simulink model "SixDsimulator_M1B"  (R2021a)
settings: Solver=FixedStepDiscrete  StartTime=0.0  StopTime=200  FixedStep=.1  RelTol=1e-3
libraries: simulink x1
settings Model: Creator=tranka  LastModifiedBy=tranka

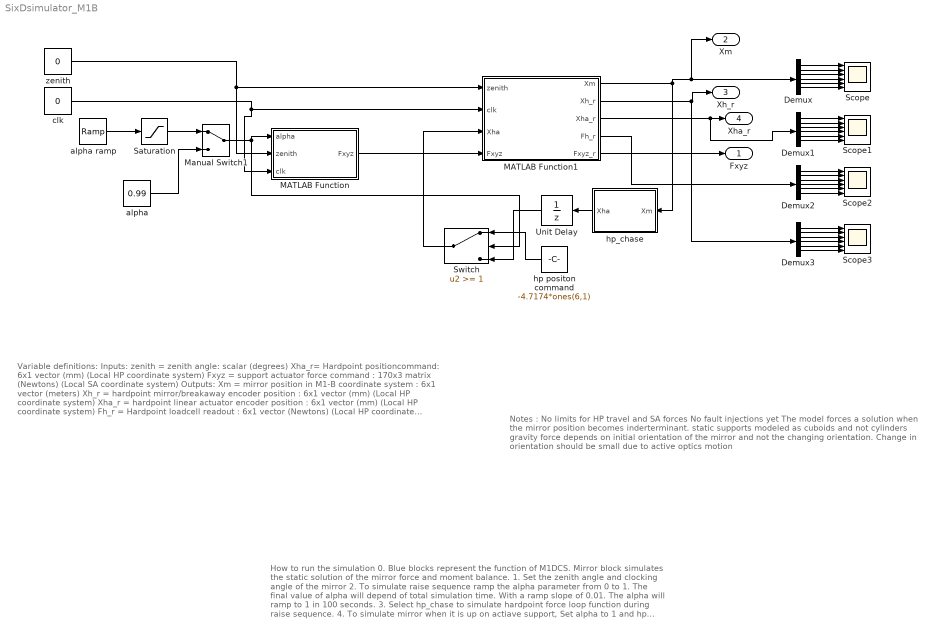
== system SixDsimulator_M1B ==
  note: How to run the simulation
      |
      | 0. Blue blocks represent the function of M1DCS. Mirror block simulates the static solution of the mirror force and moment balance.
      | 1. Set the zenith angle and clocking angle of the mirror
      | 2. To simulate raise sequence ramp the alpha parameter from 0 to 1. The final value of alpha will depend of total simulation time. With a ramp slope of 0.01. The alpha will ramp to 1 in 100 seconds.
      | 3. Select hp_chase to simulate hardpoint force loop function during raise sequence.
      | 4. To simulate mirror when it is up on actiave support, Set alpha to 1 and hp position command as user input.
  note: Variable definitions:
      |
      | Inputs:
      | zenith = zenith angle: scalar (degrees)
      | Xha_r= Hardpoint positioncommand: 6x1 vector (mm) (Local HP coordinate system)
      | Fxyz = support actuator force command : 170x3 matrix (Newtons) (Local SA coordinate system)
      |
      | Outputs:
      | Xm = mirror position in M1-B coordinate system : 6x1 vector (meters)
      | Xh_r = hardpoint mirror/breakaway encoder position : 6x1 vector (mm) (Local HP coordinate system)
      | Xha_r = hardpoint linear actuator encoder position : 6x1 vector (mm) (Local HP coordinate system)
      | Fh_r = Hardpoint loadcell readout : 6x1 vector (Newtons) (Local HP coordinate system)
      | FXYZ_r = support actuator force readback : 170x3 matrix (SA local coordinate system)
  note: Notes :
      |
      | No limits for HP travel and SA forces
      | No fault injections yet
      | The model forces a solution when the mirror position becomes inderterminant.
      | static supports modeled as cuboids and not cylinders
      | gravity force depends on initial orientation of the mirror and not the changing orientation.
      | Change in orientation should be small due to active optics motion
  Demux{,1..3} (4 alike) : Demux  Outputs=6
  MATLAB Function : MATLAB Function  TreatAsAtomicUnit=on
  MATLAB Function1 : MATLAB Function  TreatAsAtomicUnit=on
  Manual Switch1 : ManualSwitch
  Saturation : Saturate  UpperLimit=1  LowerLimit=-1
  Scope{,1..3} (4 alike) : Scope  NumInputPorts=6
  Switch : Switch  Threshold=1
  Unit Delay : UnitDelay  SampleTime=-1  HasFrameUpgradeWarning=on
  alpha : Constant  Value=0.99
  alpha ramp : simulink/Sources/Ramp  slope=0.01  start=0  InitialOutput=0
  clk : Constant  Value=0
  hp positon command : Constant  Value=-4.7174*ones(6,1)
  hp_chase : MATLAB Function  TreatAsAtomicUnit=on
  zenith : Constant  Value=0
  Fxyz : Outport
  Xm : Outport  Port=2
  Xh_r : Outport  Port=3
  Xha_r : Outport  Port=4
  wires:
  MATLAB Function/1(Fxyz) -> MATLAB Function1/4(Fxyz)
  zenith/1 -> MATLAB Function1/1(zenith), MATLAB Function/2(zenith)
  MATLAB Function1/1(Xm) -> Xm/1, Demux/1, hp_chase/1(Xm)
  hp_chase/1(Xha) -> Unit Delay/1
  Demux/3 -> Scope/3
  Demux/4 -> Scope/4
  Demux/5 -> Scope/5
  Demux/2 -> Scope/2
  Demux/6 -> Scope/6
  Demux/1 -> Scope/1
  Demux1/1 -> Scope1/1
  Demux1/2 -> Scope1/2
  Demux1/3 -> Scope1/3
  Demux1/4 -> Scope1/4
  Demux1/5 -> Scope1/5
  Demux1/6 -> Scope1/6
  MATLAB Function1/3(Xha_r) -> Demux1/1, Xha_r/1
  Demux2/1 -> Scope2/1
  Demux2/2 -> Scope2/2
  Demux2/3 -> Scope2/3
  Demux2/5 -> Scope2/5
  Demux2/6 -> Scope2/6
  Demux2/4 -> Scope2/4
  MATLAB Function1/4(Fh_r) -> Demux2/1
  alpha ramp/1 -> Saturation/1
  alpha/1 -> Manual Switch1/2
  Manual Switch1/1 -> Switch/2, MATLAB Function/1(alpha)
  clk/1 -> MATLAB Function/3(clk), MATLAB Function1/2(clk)
  MATLAB Function1/5(Fxyz_r) -> Fxyz/1
  MATLAB Function1/2(Xh_r) -> Demux3/1, Xh_r/1
  Demux3/1 -> Scope3/1
  Demux3/4 -> Scope3/4
  Demux3/2 -> Scope3/2
  Demux3/6 -> Scope3/6
  Demux3/3 -> Scope3/3
  Demux3/5 -> Scope3/5
  Saturation/1 -> Manual Switch1/1
  hp positon command/1 -> Switch/1
  Unit Delay/1 -> Switch/3
  Switch/1 -> MATLAB Function1/3(Xha)

== matlab function SixDsimulator_M1B/MATLAB Function1 ==
  data: zenith input; clk input; Xm output; Xha input; Fxyz input; Xh_r output; Xha_r output; Fh_r output; Fxyz_r output
function [Xm,Xh_r,Xha_r,Fh_r, Fxyz_r] = mirror(zenith,clk, Xha,Fxyz)
%% fix input coordinates, indexes, units etc
% pass the support actuator to output
% In future implement SA force limits or disable a few actuators.
Fxyz_r = Fxyz; 

sign_matrix = [-1    -1    -1
    -1    -1    -1
    -1    -1    -1
    -1    -1    -1
     1     1    -1
     1     1    -1
    -1    -1    -1
    -1    -1    -1
    -1    -1    -1
    -1    -1    -1
    -1    -1    -1
     1     1    -1
    -1    -1    -1
    -1    -1    -1
    -1    -1    -1
    -1    -1    -1
     1     1    -1
     1     1    -1
    -1    -1    -1
    -1    -1    -1
    -1    -1    -1
    -1    -1    -1
     1     1    -1
     1     1    -1
    -1    -1    -1
    -1    -1    -1
    -1    -1    -1
     1     1    -1
     1     1    -1
    -1    -1    -1
    -1    -1    -1
     1     1    -1
     1     1    -1
     1     1    -1
     1     1    -1
     1     1    -1
     1     1    -1
     1     1    -1
     1     1    -1
     1     1    -1
     1     1    -1
     1     1    -1
     1     1    -1
     1     1    -1
     1     1    -1
     1     1    -1
     1     1    -1
     1     1    -1
     1     1    -1
     1     1    -1
     1     1    -1
     1     1    -1
     1     1    -1
     1     1    -1
     1     1    -1
     1     1    -1
     1     1    -1
     1     1    -1
     1     1    -1
     1     1    -1
     1     1    -1
     1     1    -1
     1     1    -1
     1     1    -1
     1     1    -1
     1     1    -1
     1     1    -1
     1     1    -1
     1     1    -1
     1     1    -1
     1     1    -1
     1     1    -1
     1     1    -1
     1     1    -1
     1     1    -1
     1     1    -1
     1     1    -1
     1     1    -1
     1     1    -1
     1     1    -1
     1     1    -1
     1     1    -1
     1     1    -1
     1     1    -1
     1     1    -1
     1     1    -1
     1     1    -1
     1     1    -1
     1     1    -1
     1     1    -1
     1     1    -1
     1     1    -1
     1     1    -1
     1     1    -1
     1     1    -1
     1     1    -1
     1     1    -1
     1     1    -1
     1     1    -1
     1     1    -1
     1     1    -1
     1     1    -1
     1     1    -1
     1     1    -1
     1     1    -1
     1     1    -1
     1     1    -1
     1     1    -1
     1     1    -1
     1     1    -1
     1     1    -1
     1     1    -1
     1     1    -1
     1     1    -1
     1     1    -1
     1     1    -1
     1     1    -1
    -1    -1    -1
    -1    -1    -1
    -1    -1    -1
    -1    -1    -1
    -1    -1    -1
     1     1    -1
    -1    -1    -1
    -1    -1    -1
    -1    -1    -1
    -1    -1    -1
     1     1    -1
     1     1    -1
    -1    -1    -1
    -1    -1    -1
    -1    -1    -1
    -1    -1    -1
     1     1    -1
     1     1    -1
    -1    -1    -1
    -1    -1    -1
    -1    -1    -1
     1     1    -1
     1     1    -1
    -1    -1    -1
    -1    -1    -1
     1     1    -1
     1     1    -1
     1     1    -1
     1     1    -1
     1     1    -1
     1     1    -1
     1     1    -1
     1     1    -1
     1     1    -1
     1     1    -1
     1     1    -1
     1     1    -1
     1     1    -1
     1     1    -1
     1     1    -1
     1     1    -1
     1     1    -1
     1     1    -1
     1     1    -1
     1     1    -1
     1     1    -1
     1     1    -1
     1     1    -1
    -1    -1    -1
    -1    -1    -1
    -1    -1    -1
    -1    -1    -1
    -1    -1    -1];
Fxyz = sign_matrix.*Fxyz;
Fxyz = node_rearangement(Fxyz);
Xha = Xha*1e-3; % millimeter to meter
Xha = -Xha; % HP to M1 B coordinates

%% Constants and transforms
t = 13.5; % tilt of the off axis mirror
% clk = 60; % clocking angle of one of the off axis mirror.

% transforms
% *HP*
% HP2XYZ = [0.38460668	-0.38460668	0.07381907	0.4584258	-0.4584258	-0.07381907;
% 0.30761081	0.30761081	-0.48640517	0.17975252	0.17975252	-0.48640517;
% 0.22921984	0.22921984	0.23032414	0.2293977	0.2293977	0.23032414;
% -0.10285998	-0.10285998	-0.05037601	0.153236	0.153236	-0.05037601;
% -0.11744075	0.11744075	0.14797153	0.03018701	-0.03018701	-0.14797153;
% 0.08255542	-0.08255542	0.08218629	-0.08243407	0.08243407	-0.08218629];

% position M1B to HP coordinate system
XYZ2HP = [-0.45302	0.517744	-0.72575	1.934433	-1.14293	-2.02285;
0.453021	0.517744	-0.72575	1.934433	1.14293	2.02285;
-0.22187	-0.6512	-0.72575	0.02259	2.246733	-2.02285;
-0.67489	0.133456	-0.72575	-1.95702	1.103803	2.02285;
0.67489	0.133456	-0.72575	-1.95702	-1.1038	-2.02285;
0.221869	-0.6512	-0.72575	0.02259	-2.24673	2.02285];

H = -XYZ2HP; %M1B XYZ to M1B HP

% force
HP2XYZ = [-0.45302	0.45302	-0.22187	-0.67489	0.67489	0.22187
0.51774	0.51774	-0.65120	0.13346	0.13346	-0.65120
-0.72575	-0.72575	-0.72575	-0.72575	-0.72575	-0.72575
1.93443	1.93443	0.02259	-1.95702	-1.95702	0.02259
-1.14293	1.14293	2.24673	1.10380	-1.10380	-2.24673
-2.02285	2.02285	-2.02285	2.02285	-2.02285	2.02285];

Th = -HP2XYZ;


% *Equivalent static supports SS*
% Ks_eq = 2.5e5*110; % equivalent static support stiffness
X_ss_gap = [8e-3 8e-3 6.5e-3 8e-3 8e-3 6.5e-3 8e-3 8e-3 6.5e-3]';
% Xm_gap = [8e-3 8e-3 6.5e-3 0 0 0]';

sr1y = 3; sr1x = 0;
sr2x = 3*cosd(210);sr2y = 3*sind(210);
sr3x = 3*cosd(330);sr3y = 3*sind(330);

S2M = [1 0 0 1 0 0 1 0 0;
         0 1 0 0 1 0 0 1 0;
         0 0 1 0 0 1 0 0 1;
         0 0 sr1y 0 0 sr2y 0 0 sr3y;
         0 0 -sr1x 0 0 -sr2x 0 0 -sr3x;
         -sr1y sr1x 0 -sr2y sr2x 0 -sr3y sr3x 0];
% M2S = pinv(S2M);
Ts =     S2M;
ds2dm = [1/3 0 0 1/3 0 0 1/3 0 0;
         0 1/3 0 0 1/3 0 0 1/3 0;
         0 0 1/3 0 0 1/3 0 0 1/3;
         0 0 sr1y 0 0 sr2y 0 0 sr3y;
         0 0 -sr1x 0 0 -sr2x 0 0 -sr3x;
         -sr1y sr1x  0 -sr2y sr2x 0 -sr3y sr3x 0];
S = pinv(ds2dm);
% Ts = ds2dm;

%% persistent variables
persistent Fa_prev  Xm_prev;
% persistent Xha_prev;


if isempty(Fa_prev)
    Fa_prev = zeros(6,1);
end



%% initial down condition

[~, ~, FMg] = decompose_gravity_vector(t,clk,zenith); % decompose gravity vector

if isempty(Xm_prev)
    Fss = Force_M2S(-(FMg+Fa_prev)); % static support reaction force
    Xs = ss_compression_tension(Fss); % static support compression/tension under mirror weight
    Xs = Xs + sign(Xs).*X_ss_gap;
    Xm_prev = Slength2Mlength(Xs); % mirror position 
    Xs0 = sign(Xs).*X_ss_gap;
    Xha = dm2dh(Slength2Mlength(Xs0));
end
if isempty(Xha)
    Xha = dm2dh(Slength2Mlength(Xs0));
end

%% static support stiffness update

Xs = Mlength2Slength(Xm_prev); % mirror position at equivalent static supports
Ks = ss_stiffness(Xs);

%% Support actuator force and moment applied

FMa = ActForces2FM(Fxyz);

%% hardpoint force due to motion of hardpoint actuator only
% during chase
Xh_r = dm2dh(Xm_prev);
[~, Kh, Fhbk] = hp_stiffness(Xh_r,Xha);

% after chase
if (FMg+FMa) < 100 
    Kh = 120e6*eye(6);
    Fhbk = zeros(6,1);
end

%% new mirror position to to support actuator force update
% Xm in M1B
Xm = pinv(Ts*Ks*S + Th*Kh*H)*(FMg + FMa + Ts*Ks*(sign(Xs).*X_ss_gap) + Th*Kh*Xha + Th*Fhbk );


%% hardopint reaction force and mirror encoder update
Xh_r = dm2dh(Xm);
[Fh_r, ~, ~] = hp_stiffness(Xh_r,Xha);

%% update variables for simulation and outputs except Fxyz
Fa_prev = FMa;
Xm_prev = Xm; % in M1B
% Fxyz_r = sign_matrix.*Fxyz; % change it to local actuator coordinate system
% Fxyz_r = Fxyz;
Xha_r = -Xha*1e3; % change it to HP coordinate system and mm
Xh_r = -Xh_r*1e3; % change it to HP coordinate system and mm

== matlab function SixDsimulator_M1B/MATLAB Function ==
  data: alpha input; Fxyz output; zenith input; clk input
function Fxyz  = Act_forces(alpha,zenith,clk)
t = 13.5; % tilt of the off axis mirror
% clk = 60; % clocking angle of one of the off axis mirror.
% zenith = 30;
% alpha = 1;
[Fg, FM, FMg] = decompose_gravity_vector(t,clk,zenith);

FM = alpha*FMg;

K = [    0         0         0         0         0         0;
         0         0         0         0         0         0;
    0.0004    0.0013   -0.0056    0.0049    0.0013         0;
   -0.0115         0         0         0         0   -0.0026;
         0   -0.0115         0         0         0   -0.0043;
    0.0010    0.0005   -0.0066    0.0015    0.0025         0;
   -0.0115         0         0         0         0    0.0026;
         0   -0.0115         0         0         0   -0.0043;
    0.0009   -0.0005   -0.0066   -0.0015    0.0025         0;
   -0.0115         0         0         0         0   -0.0026;
         0   -0.0115         0         0         0    0.0043;
   -0.0010    0.0005   -0.0066    0.0015   -0.0025         0;
   -0.0115         0         0         0         0    0.0026;
         0   -0.0115         0         0         0    0.0043;
   -0.0009   -0.0005   -0.0066   -0.0015   -0.0025         0;
         0         0         0         0         0         0;
         0         0         0         0         0         0;
   -0.0010    0.0006   -0.0020    0.0007    0.0043         0;
         0         0         0         0         0         0;
         0         0         0         0         0         0;
   -0.0011   -0.0005   -0.0020   -0.0007    0.0043         0;
         0         0         0         0         0         0;
         0         0         0         0         0         0;
    0.0010   -0.0002   -0.0058   -0.0007    0.0047         0;
         0         0         0         0         0         0;
         0         0         0         0         0         0;
    0.0009    0.0002   -0.0058    0.0007    0.0047         0;
         0         0         0         0         0         0;
         0         0         0         0         0         0;
    0.0010    0.0006   -0.0020    0.0007   -0.0043         0;
         0         0         0         0         0         0;
         0         0         0         0         0         0;
    0.0011   -0.0005   -0.0020   -0.0007   -0.0043         0;
         0         0         0         0         0         0;
         0         0         0         0         0         0;
   -0.0010   -0.0002   -0.0058   -0.0007   -0.0047         0;
         0         0         0         0         0         0;
         0         0         0         0         0         0;
   -0.0009    0.0001   -0.0058    0.0007   -0.0047         0;
         0         0         0         0         0         0;
         0         0         0         0         0         0;
   -0.0005   -0.0006   -0.0030   -0.0039   -0.0030         0;
         0         0         0         0         0         0;
         0         0         0         0         0         0;
    0.0001    0.0005   -0.0047   -0.0035   -0.0029         0;
         0         0         0         0         0         0;
         0         0         0         0         0         0;
    0.0005   -0.0006   -0.0030   -0.0039    0.0030         0;
         0         0         0         0         0         0;
         0         0         0         0         0         0;
   -0.0001    0.0005   -0.0047   -0.0035    0.0029         0;
         0         0         0         0         0         0;
         0         0         0         0         0         0;
   -0.0005    0.0006   -0.0030    0.0039   -0.0030         0;
         0         0         0         0         0         0;
         0         0         0         0         0         0;
    0.0001   -0.0005   -0.0047    0.0035   -0.0029         0;
         0         0         0         0         0         0;
         0         0         0         0         0         0;
    0.0005    0.0006   -0.0030    0.0039    0.0030         0;
         0         0         0         0         0         0;
         0         0         0         0         0         0;
   -0.0001   -0.0005   -0.0047    0.0035    0.0029         0;
         0         0         0         0         0         0;
         0         0         0         0         0         0;
   -0.0003    0.0014   -0.0068   -0.0044    0.0003         0;
         0         0         0         0         0         0;
         0         0         0         0         0         0;
    0.0000    0.0017   -0.0070   -0.0044    0.0011         0;
         0         0         0         0         0         0;
         0         0         0         0         0         0;
   -0.0004    0.0018   -0.0064   -0.0036    0.0021         0;
         0         0         0         0         0         0;
         0         0         0         0         0         0;
   -0.0016    0.0012   -0.0067   -0.0029    0.0033         0;
         0         0         0         0         0         0;
         0         0         0         0         0         0;
   -0.0017    0.0007   -0.0070   -0.0022    0.0037         0;
         0         0         0         0         0         0;
         0         0         0         0         0         0;
   -0.0014    0.0016   -0.0067   -0.0015    0.0041         0;
         0         0         0         0         0         0;
         0         0         0         0         0         0;
   -0.0013    0.0001   -0.0068   -0.0000    0.0041         0;
         0         0         0         0         0         0;
         0         0         0         0         0         0;
   -0.0003   -0.0013   -0.0067    0.0044    0.0003         0;
         0         0         0         0         0         0;
         0         0         0         0         0         0;
   -0.0000   -0.0016   -0.0069    0.0044    0.0011         0;
         0         0         0         0         0         0;
         0         0         0         0         0         0;
   -0.0005   -0.0017   -0.0064    0.0036    0.0021         0;
         0         0         0         0         0         0;
         0         0         0         0         0         0;
   -0.0016   -0.0012   -0.0067    0.0029    0.0033         0;
         0         0         0         0         0         0;
         0         0         0         0         0         0;
   -0.0017   -0.0007   -0.0070    0.0022    0.0037         0;
         0         0         0         0         0         0;
         0         0         0         0         0         0;
   -0.0014   -0.0015   -0.0066    0.0015    0.0041         0;
         0         0         0         0         0         0;
         0         0         0         0         0         0;
    0.0003    0.0014   -0.0068   -0.0044   -0.0003         0;
         0         0         0         0         0         0;
         0         0         0         0         0         0;
   -0.0000    0.0017   -0.0070   -0.0044   -0.0011         0;
         0         0         0         0         0         0;
         0         0         0         0         0         0;
    0.0004    0.0018   -0.0064   -0.0036   -0.0021         0;
         0         0         0         0         0         0;
         0         0         0         0         0         0;
    0.0016    0.0012   -0.0067   -0.0029   -0.0033         0;
         0         0         0         0         0         0;
         0         0         0         0         0         0;
    0.0017    0.0007   -0.0070   -0.0022   -0.0037         0;
         0         0         0         0         0         0;
         0         0         0         0         0         0;
    0.0014    0.0016   -0.0067   -0.0015   -0.0041         0;
         0         0         0         0         0         0;
         0         0         0         0         0         0;
    0.0013    0.0001   -0.0068   -0.0000   -0.0041         0;
         0         0         0         0         0         0;
         0         0         0         0         0         0;
    0.0003   -0.0013   -0.0067    0.0044   -0.0003         0;
         0         0         0         0         0         0;
         0         0         0         0         0         0;
    0.0000   -0.0016   -0.0069    0.0044   -0.0011         0;
         0         0         0         0         0         0;
         0         0         0         0         0         0;
    0.0005   -0.0017   -0.0064    0.0036   -0.0021         0;
         0         0         0         0         0         0;
         0         0         0         0         0         0;
    0.0016   -0.0012   -0.0067    0.0029   -0.0033         0;
         0         0         0         0         0         0;
         0         0         0         0         0         0;
    0.0017   -0.0007   -0.0070    0.0022   -0.0037         0;
         0         0         0         0         0         0;
         0         0         0         0         0         0;
    0.0014   -0.0015   -0.0066    0.0015   -0.0041         0;
         0         0         0         0         0         0;
         0         0         0         0         0         0;
    0.0004   -0.0007   -0.0031   -0.0047    0.0019         0;
         0         0         0         0         0         0;
         0         0         0         0         0         0;
    0.0014   -0.0003   -0.0024   -0.0013    0.0047         0;
         0         0         0         0         0         0;
         0         0         0         0         0         0;
    0.0004    0.0007   -0.0031    0.0047    0.0019         0;
         0         0         0         0         0         0;
         0         0         0         0         0         0;
    0.0013    0.0002   -0.0024    0.0013    0.0047         0;
         0         0         0         0         0         0;
         0         0         0         0         0         0;
    0.0004   -0.0019   -0.0061   -0.0051    0.0004         0;
         0         0         0         0         0         0;
         0         0         0         0         0         0;
    0.0004   -0.0014   -0.0056   -0.0049    0.0013         0;
         0         0         0         0         0         0;
         0         0         0         0         0         0;
    0.0007   -0.0016   -0.0060   -0.0043    0.0025         0;
         0         0         0         0         0         0;
         0         0         0         0         0         0;
    0.0013   -0.0011   -0.0048   -0.0035    0.0035         0;
         0         0         0         0         0         0;
         0         0         0         0         0         0;
    0.0009   -0.0006   -0.0059   -0.0027    0.0041         0;
         0         0         0         0         0         0;
         0         0         0         0         0         0;
   -0.0004    0.0002   -0.0039   -0.0041    0.0019         0;
         0         0         0         0         0         0;
         0         0         0         0         0         0;
    0.0014   -0.0005   -0.0055   -0.0019    0.0045         0;
         0         0         0         0         0         0;
         0         0         0         0         0         0;
    0.0008   -0.0000   -0.0056   -0.0000    0.0048         0;
         0         0         0         0         0         0;
         0         0         0         0         0         0;
    0.0004    0.0018   -0.0061    0.0051    0.0004         0;
         0         0         0         0         0         0;
         0         0         0         0         0         0;
    0.0007    0.0015   -0.0060    0.0043    0.0025         0;
         0         0         0         0         0         0;
         0         0         0         0         0         0;
    0.0013    0.0011   -0.0048    0.0035    0.0035         0;
         0         0         0         0         0         0;
         0         0         0         0         0         0;
    0.0009    0.0006   -0.0059    0.0027    0.0041         0;
         0         0         0         0         0         0;
         0         0         0         0         0         0;
   -0.0004   -0.0002   -0.0038    0.0041    0.0019         0;
         0         0         0         0         0         0;
         0         0         0         0         0         0;
    0.0013    0.0005   -0.0055    0.0019    0.0045         0;
   -0.0127         0         0         0         0    0.0013;
         0   -0.0128         0         0         0   -0.0009;
    0.0015   -0.0003   -0.0063   -0.0007    0.0005         0;
   -0.0116         0         0         0         0    0.0039;
         0   -0.0116         0         0         0   -0.0009;
    0.0009   -0.0003   -0.0066   -0.0022    0.0005         0;
   -0.0113         0         0         0         0    0.0066;
         0   -0.0113         0         0         0   -0.0009;
    0.0012    0.0014   -0.0071   -0.0036    0.0005         0;
   -0.0118         0         0         0         0    0.0026;
         0   -0.0118         0         0         0   -0.0016;
    0.0004   -0.0002   -0.0058   -0.0015    0.0009         0;
   -0.0114         0         0         0         0    0.0053;
         0   -0.0114         0         0         0   -0.0016;
    0.0006   -0.0008   -0.0060   -0.0029    0.0009         0;
   -0.0115         0         0         0         0    0.0039;
         0   -0.0115         0         0         0   -0.0023;
    0.0006   -0.0012   -0.0066   -0.0022    0.0013         0;
   -0.0113         0         0         0         0    0.0066;
         0   -0.0113         0         0         0   -0.0023;
   -0.0014    0.0013   -0.0071   -0.0036    0.0013         0;
   -0.0117         0         0         0         0    0.0026;
         0   -0.0117         0         0         0   -0.0029;
    0.0006   -0.0003   -0.0065   -0.0015    0.0017         0;
   -0.0114         0         0         0         0    0.0053;
         0   -0.0114         0         0         0   -0.0029;
   -0.0001    0.0003   -0.0069   -0.0029    0.0017         0;
   -0.0115         0         0         0         0    0.0039;
         0   -0.0115         0         0         0   -0.0036;
    0.0008   -0.0005   -0.0064   -0.0022    0.0021         0;
   -0.0114         0         0         0         0    0.0053;
         0   -0.0114         0         0         0   -0.0043;
   -0.0012    0.0016   -0.0072   -0.0029    0.0025         0;
   -0.0114         0         0         0         0    0.0039;
         0   -0.0114         0         0         0   -0.0050;
   -0.0013    0.0006   -0.0069   -0.0022    0.0029         0;
   -0.0115         0         0         0         0    0.0026;
         0   -0.0115         0         0         0   -0.0056;
   -0.0014    0.0006   -0.0067   -0.0015    0.0033         0;
   -0.0122         0         0         0         0    0.0013;
         0   -0.0121         0         0         0   -0.0023;
    0.0003   -0.0002   -0.0063   -0.0007    0.0013         0;
   -0.0118         0         0         0         0    0.0013;
         0   -0.0118         0         0         0   -0.0036;
    0.0009   -0.0003   -0.0063   -0.0007    0.0021         0;
   -0.0132         0         0         0         0   -0.0000;
         0   -0.0131         0         0         0   -0.0016;
    0.0009   -0.0000   -0.0057    0.0000    0.0009         0;
   -0.0121         0         0         0         0   -0.0000;
         0   -0.0121         0         0         0   -0.0029;
    0.0002   -0.0000   -0.0064    0.0000    0.0017         0;
   -0.0116         0         0         0         0    0.0013;
         0   -0.0116         0         0         0   -0.0050;
    0.0005   -0.0002   -0.0066   -0.0007    0.0029         0;
   -0.0115         0         0         0         0    0.0013;
         0   -0.0115         0         0         0   -0.0063;
   -0.0014    0.0000   -0.0072   -0.0007    0.0037         0;
   -0.0117         0         0         0         0    0.0000;
         0   -0.0117         0         0         0   -0.0043;
    0.0012   -0.0000   -0.0065   -0.0000    0.0025         0;
   -0.0115         0         0         0         0   -0.0000;
         0   -0.0115         0         0         0   -0.0056;
   -0.0008   -0.0000   -0.0067    0.0000    0.0033         0;
   -0.0127         0         0         0         0   -0.0013;
         0   -0.0128         0         0         0   -0.0009;
    0.0015    0.0003   -0.0063    0.0007    0.0005         0;
   -0.0115         0         0         0         0   -0.0039;
         0   -0.0116         0         0         0   -0.0009;
    0.0008    0.0004   -0.0065    0.0022    0.0005         0;
   -0.0113         0         0         0         0   -0.0066;
         0   -0.0113         0         0         0   -0.0009;
    0.0011   -0.0014   -0.0071    0.0036    0.0005         0;
   -0.0118         0         0         0         0   -0.0026;
         0   -0.0118         0         0         0   -0.0016;
    0.0004    0.0002   -0.0057    0.0015    0.0009         0;
   -0.0114         0         0         0         0   -0.0053;
         0   -0.0114         0         0         0   -0.0016;
    0.0006    0.0009   -0.0060    0.0029    0.0009         0;
   -0.0115         0         0         0         0   -0.0039;
         0   -0.0115         0         0         0   -0.0023;
    0.0006    0.0012   -0.0066    0.0022    0.0013         0;
   -0.0113         0         0         0         0   -0.0066;
         0   -0.0113         0         0         0   -0.0023;
   -0.0014   -0.0013   -0.0070    0.0036    0.0013         0;
   -0.0117         0         0         0         0   -0.0026;
         0   -0.0117         0         0         0   -0.0029;
    0.0006    0.0003   -0.0065    0.0015    0.0017         0;
   -0.0114         0         0         0         0   -0.0053;
         0   -0.0114         0         0         0   -0.0029;
   -0.0001   -0.0003   -0.0068    0.0029    0.0017         0;
   -0.0114         0         0         0         0   -0.0039;
         0   -0.0115         0         0         0   -0.0036;
    0.0008    0.0005   -0.0064    0.0022    0.0021         0;
   -0.0113         0         0         0         0   -0.0053;
         0   -0.0113         0         0         0   -0.0043;
   -0.0012   -0.0016   -0.0072    0.0029    0.0025         0;
   -0.0114         0         0         0         0   -0.0039;
         0   -0.0114         0         0         0   -0.0050;
   -0.0013   -0.0006   -0.0068    0.0022    0.0029         0;
   -0.0114         0         0         0         0   -0.0026;
         0   -0.0115         0         0         0   -0.0056;
   -0.0013   -0.0006   -0.0067    0.0015    0.0033         0;
   -0.0122         0         0         0         0   -0.0013;
         0   -0.0121         0         0         0   -0.0023;
    0.0003    0.0001   -0.0063    0.0007    0.0013         0;
   -0.0118         0         0         0         0   -0.0013;
         0   -0.0118         0         0         0   -0.0036;
    0.0009    0.0003   -0.0063    0.0007    0.0021         0;
   -0.0116         0         0         0         0   -0.0013;
         0   -0.0116         0         0         0   -0.0050;
    0.0005    0.0002   -0.0066    0.0007    0.0029         0;
   -0.0115         0         0         0         0   -0.0013;
         0   -0.0115         0         0         0   -0.0063;
   -0.0014    0.0000   -0.0072    0.0007    0.0037         0;
   -0.0135         0         0         0         0   -0.0000;
         0   -0.0135         0         0         0         0;
    0.0000   -0.0000   -0.0102    0.0000         0         0;
   -0.0135         0         0         0         0    0.0026;
         0   -0.0135         0         0         0         0;
    0.0000   -0.0009   -0.0104   -0.0015         0         0;
   -0.0135         0         0         0         0    0.0053;
         0   -0.0135         0         0         0         0;
   -0.0000   -0.0010   -0.0110   -0.0029         0         0;
   -0.0135         0         0         0         0   -0.0026;
         0   -0.0135         0         0         0         0;
   -0.0000    0.0009   -0.0104    0.0015         0         0;
   -0.0135         0         0         0         0   -0.0053;
         0   -0.0135         0         0         0         0;
   -0.0000    0.0010   -0.0109    0.0029         0         0;
         0         0         0         0         0         0;
         0         0         0         0         0         0;
   -0.0004   -0.0007   -0.0031   -0.0047   -0.0019         0;
         0         0         0         0         0         0;
         0         0         0         0         0         0;
   -0.0014   -0.0003   -0.0024   -0.0013   -0.0047         0;
         0         0         0         0         0         0;
         0         0         0         0         0         0;
   -0.0004    0.0007   -0.0031    0.0047   -0.0019         0;
         0         0         0         0         0         0;
         0         0         0         0         0         0;
   -0.0014    0.0002   -0.0024    0.0013   -0.0047         0;
         0         0         0         0         0         0;
         0         0         0         0         0         0;
   -0.0004   -0.0019   -0.0061   -0.0051   -0.0004         0;
         0         0         0         0         0         0;
         0         0         0         0         0         0;
   -0.0004   -0.0014   -0.0056   -0.0049   -0.0013         0;
         0         0         0         0         0         0;
         0         0         0         0         0         0;
   -0.0007   -0.0016   -0.0060   -0.0043   -0.0025         0;
         0         0         0         0         0         0;
         0         0         0         0         0         0;
   -0.0013   -0.0011   -0.0048   -0.0035   -0.0035         0;
         0         0         0         0         0         0;
         0         0         0         0         0         0;
   -0.0009   -0.0006   -0.0059   -0.0027   -0.0041         0;
         0         0         0         0         0         0;
         0         0         0         0         0         0;
    0.0004    0.0002   -0.0039   -0.0041   -0.0019         0;
         0         0         0         0         0         0;
         0         0         0         0         0         0;
   -0.0014   -0.0005   -0.0055   -0.0019   -0.0045         0;
         0         0         0         0         0         0;
         0         0         0         0         0         0;
   -0.0008   -0.0000   -0.0056   -0.0000   -0.0048         0;
         0         0         0         0         0         0;
         0         0         0         0         0         0;
   -0.0004    0.0018   -0.0061    0.0051   -0.0004         0;
         0         0         0         0         0         0;
         0         0         0         0         0         0;
   -0.0004    0.0013   -0.0056    0.0049   -0.0013         0;
         0         0         0         0         0         0;
         0         0         0         0         0         0;
   -0.0007    0.0015   -0.0060    0.0043   -0.0025         0;
         0         0         0         0         0         0;
         0         0         0         0         0         0;
   -0.0013    0.0011   -0.0048    0.0035   -0.0035         0;
         0         0         0         0         0         0;
         0         0         0         0         0         0;
   -0.0009    0.0006   -0.0059    0.0027   -0.0041         0;
         0         0         0         0         0         0;
         0         0         0         0         0         0;
    0.0004   -0.0002   -0.0038    0.0041   -0.0019         0;
         0         0         0         0         0         0;
         0         0         0         0         0         0;
   -0.0013    0.0005   -0.0055    0.0019   -0.0045         0;
   -0.0127         0         0         0         0    0.0013;
         0   -0.0128         0         0         0    0.0009;
   -0.0015   -0.0003   -0.0063   -0.0007   -0.0005         0;
   -0.0116         0         0         0         0    0.0039;
         0   -0.0116         0         0         0    0.0009;
   -0.0009   -0.0003   -0.0066   -0.0022   -0.0005         0;
   -0.0113         0         0         0         0    0.0066;
         0   -0.0113         0         0         0    0.0009;
   -0.0012    0.0014   -0.0071   -0.0036   -0.0005         0;
   -0.0118         0         0         0         0    0.0026;
         0   -0.0118         0         0         0    0.0016;
   -0.0004   -0.0002   -0.0058   -0.0015   -0.0009         0;
   -0.0114         0         0         0         0    0.0053;
         0   -0.0114         0         0         0    0.0016;
   -0.0006   -0.0008   -0.0060   -0.0029   -0.0009         0;
   -0.0115         0         0         0         0    0.0039;
         0   -0.0115         0         0         0    0.0023;
   -0.0006   -0.0012   -0.0066   -0.0022   -0.0013         0;
   -0.0113         0         0         0         0    0.0066;
         0   -0.0113         0         0         0    0.0023;
    0.0014    0.0013   -0.0071   -0.0036   -0.0013         0;
   -0.0117         0         0         0         0    0.0026;
         0   -0.0117         0         0         0    0.0029;
   -0.0006   -0.0003   -0.0065   -0.0015   -0.0017         0;
   -0.0114         0         0         0         0    0.0053;
         0   -0.0114         0         0         0    0.0029;
    0.0001    0.0003   -0.0069   -0.0029   -0.0017         0;
   -0.0115         0         0         0         0    0.0039;
         0   -0.0115         0         0         0    0.0036;
   -0.0008   -0.0005   -0.0064   -0.0022   -0.0021         0;
   -0.0114         0         0         0         0    0.0053;
         0   -0.0114         0         0         0    0.0043;
    0.0012    0.0016   -0.0072   -0.0029   -0.0025         0;
   -0.0114         0         0         0         0    0.0039;
         0   -0.0114         0         0         0    0.0050;
    0.0013    0.0006   -0.0069   -0.0022   -0.0029         0;
   -0.0115         0         0         0         0    0.0026;
         0   -0.0115         0         0         0    0.0056;
    0.0014    0.0006   -0.0067   -0.0015   -0.0033         0;
   -0.0122         0         0         0         0    0.0013;
         0   -0.0121         0         0         0    0.0023;
   -0.0003   -0.0002   -0.0063   -0.0007   -0.0013         0;
   -0.0118         0         0         0         0    0.0013;
         0   -0.0118         0         0         0    0.0036;
   -0.0009   -0.0003   -0.0063   -0.0007   -0.0021         0;
   -0.0132         0         0         0         0   -0.0000;
         0   -0.0131         0         0         0    0.0016;
   -0.0009   -0.0000   -0.0057    0.0000   -0.0009         0;
   -0.0121         0         0         0         0   -0.0000;
         0   -0.0121         0         0         0    0.0029;
   -0.0002   -0.0000   -0.0064    0.0000   -0.0017         0;
   -0.0116         0         0         0         0    0.0013;
         0   -0.0116         0         0         0    0.0050;
   -0.0005   -0.0002   -0.0066   -0.0007   -0.0029         0;
   -0.0115         0         0         0         0    0.0013;
         0   -0.0115         0         0         0    0.0063;
    0.0014    0.0000   -0.0072   -0.0007   -0.0037         0;
   -0.0118         0         0         0         0    0.0000;
         0   -0.0117         0         0         0    0.0043;
   -0.0012   -0.0000   -0.0065   -0.0000   -0.0025         0;
   -0.0115         0         0         0         0   -0.0000;
         0   -0.0115         0         0         0    0.0056;
    0.0008   -0.0000   -0.0067    0.0000   -0.0033         0;
   -0.0127         0         0         0         0   -0.0013;
         0   -0.0128         0         0         0    0.0009;
   -0.0015    0.0003   -0.0063    0.0007   -0.0005         0;
   -0.0115         0         0         0         0   -0.0039;
         0   -0.0116         0         0         0    0.0009;
   -0.0008    0.0004   -0.0065    0.0022   -0.0005         0;
   -0.0113         0         0         0         0   -0.0066;
         0   -0.0113         0         0         0    0.0009;
   -0.0011   -0.0014   -0.0071    0.0036   -0.0005         0;
   -0.0118         0         0         0         0   -0.0026;
         0   -0.0118         0         0         0    0.0016;
   -0.0004    0.0002   -0.0057    0.0015   -0.0009         0;
   -0.0114         0         0         0         0   -0.0053;
         0   -0.0114         0         0         0    0.0016;
   -0.0006    0.0009   -0.0060    0.0029   -0.0009         0;
   -0.0115         0         0         0         0   -0.0039;
         0   -0.0115         0         0         0    0.0023;
   -0.0006    0.0012   -0.0066    0.0022   -0.0013         0;
   -0.0113         0         0         0         0   -0.0066;
         0   -0.0113         0         0         0    0.0023;
    0.0014   -0.0013   -0.0070    0.0036   -0.0013         0;
   -0.0117         0         0         0         0   -0.0026;
         0   -0.0117         0         0         0    0.0029;
   -0.0006    0.0003   -0.0065    0.0015   -0.0017         0;
   -0.0114         0         0         0         0   -0.0053;
         0   -0.0114         0         0         0    0.0029;
    0.0001   -0.0003   -0.0068    0.0029   -0.0017         0;
   -0.0114         0         0         0         0   -0.0039;
         0   -0.0115         0         0         0    0.0036;
   -0.0008    0.0005   -0.0064    0.0022   -0.0021         0;
   -0.0113         0         0         0         0   -0.0053;
         0   -0.0113         0         0         0    0.0043;
    0.0012   -0.0016   -0.0072    0.0029   -0.0025         0;
   -0.0114         0         0         0         0   -0.0039;
         0   -0.0114         0         0         0    0.0050;
    0.0013   -0.0006   -0.0068    0.0022   -0.0029         0;
   -0.0057         0         0         0         0   -0.0013;
         0   -0.0057         0         0         0    0.0028;
    0.0007   -0.0003   -0.0033    0.0007   -0.0017         0;
   -0.0061         0         0         0         0   -0.0007;
         0   -0.0061         0         0         0    0.0011;
   -0.0002    0.0001   -0.0032    0.0004   -0.0007         0;
   -0.0059         0         0         0         0   -0.0007;
         0   -0.0059         0         0         0    0.0018;
   -0.0005    0.0002   -0.0031    0.0004   -0.0011         0;
   -0.0058         0         0         0         0   -0.0007;
         0   -0.0058         0         0         0    0.0025;
   -0.0003    0.0001   -0.0033    0.0004   -0.0015         0;
   -0.0057         0         0         0         0   -0.0007;
         0   -0.0057         0         0         0    0.0032;
    0.0007    0.0000   -0.0036    0.0004   -0.0019         0;
   -0.0057         0         0         0         0   -0.0013;
         0   -0.0057         0         0         0    0.0028;
    0.0007   -0.0003   -0.0033    0.0007   -0.0017         0;
   -0.0061         0         0         0         0   -0.0007;
         0   -0.0061         0         0         0    0.0011;
   -0.0002    0.0001   -0.0032    0.0004   -0.0007         0;
   -0.0059         0         0         0         0   -0.0007;
         0   -0.0059         0         0         0    0.0018;
   -0.0005    0.0002   -0.0031    0.0004   -0.0011         0;
   -0.0058         0         0         0         0   -0.0007;
         0   -0.0058         0         0         0    0.0025;
   -0.0003    0.0001   -0.0033    0.0004   -0.0015         0;
   -0.0057         0         0         0         0   -0.0007;
         0   -0.0057         0         0         0    0.0032;
    0.0007    0.0000   -0.0036    0.0004   -0.0019         0];






%% calculate the forces at actuators when no actuators have failed.
Fxyz_d = K*FM;
nc = size(FM,2);
na = 170;
Fxyz_v = reshape(Fxyz_d,[3,na])';
Fxyz = reshape(Fxyz_v,[na*nc,3]);
sign_matrix = [-1    -1    -1
    -1    -1    -1
    -1    -1    -1
    -1    -1    -1
     1     1    -1
     1     1    -1
    -1    -1    -1
    -1    -1    -1
    -1    -1    -1
    -1    -1    -1
    -1    -1    -1
     1     1    -1
    -1    -1    -1
    -1    -1    -1
    -1    -1    -1
    -1    -1    -1
     1     1    -1
     1     1    -1
    -1    -1    -1
    -1    -1    -1
    -1    -1    -1
    -1    -1    -1
     1     1    -1
     1     1    -1
    -1    -1    -1
    -1    -1    -1
    -1    -1    -1
     1     1    -1
     1     1    -1
    -1    -1    -1
    -1    -1    -1
     1     1    -1
     1     1    -1
     1     1    -1
     1     1    -1
     1     1    -1
     1     1    -1
     1     1    -1
     1     1    -1
     1     1    -1
     1     1    -1
     1     1    -1
     1     1    -1
     1     1    -1
     1     1    -1
     1     1    -1
     1     1    -1
     1     1    -1
     1     1    -1
     1     1    -1
     1     1    -1
     1     1    -1
     1     1    -1
     1     1    -1
     1     1    -1
     1     1    -1
     1     1    -1
     1     1    -1
     1     1    -1
     1     1    -1
     1     1    -1
     1     1    -1
     1     1    -1
     1     1    -1
     1     1    -1
     1     1    -1
     1     1    -1
     1     1    -1
     1     1    -1
     1     1    -1
     1     1    -1
     1     1    -1
     1     1    -1
     1     1    -1
     1     1    -1
     1     1    -1
     1     1    -1
     1     1    -1
     1     1    -1
     1     1    -1
     1     1    -1
     1     1    -1
     1     1    -1
     1     1    -1
     1     1    -1
     1     1    -1
     1     1    -1
     1     1    -1
     1     1    -1
     1     1    -1
     1     1    -1
     1     1    -1
     1     1    -1
     1     1    -1
     1     1    -1
     1     1    -1
     1     1    -1
     1     1    -1
     1     1    -1
     1     1    -1
     1     1    -1
     1     1    -1
     1     1    -1
     1     1    -1
     1     1    -1
     1     1    -1
     1     1    -1
     1     1    -1
     1     1    -1
     1     1    -1
     1     1    -1
     1     1    -1
     1     1    -1
     1     1    -1
     1     1    -1
     1     1    -1
     1     1    -1
    -1    -1    -1
    -1    -1    -1
    -1    -1    -1
    -1    -1    -1
    -1    -1    -1
     1     1    -1
    -1    -1    -1
    -1    -1    -1
    -1    -1    -1
    -1    -1    -1
     1     1    -1
     1     1    -1
    -1    -1    -1
    -1    -1    -1
    -1    -1    -1
    -1    -1    -1
     1     1    -1
     1     1    -1
    -1    -1    -1
    -1    -1    -1
    -1    -1    -1
     1     1    -1
     1     1    -1
    -1    -1    -1
    -1    -1    -1
     1     1    -1
     1     1    -1
     1     1    -1
     1     1    -1
     1     1    -1
     1     1    -1
     1     1    -1
     1     1    -1
     1     1    -1
     1     1    -1
     1     1    -1
     1     1    -1
     1     1    -1
     1     1    -1
     1     1    -1
     1     1    -1
     1     1    -1
     1     1    -1
     1     1    -1
     1     1    -1
     1     1    -1
     1     1    -1
     1     1    -1
    -1    -1    -1
    -1    -1    -1
    -1    -1    -1
    -1    -1    -1
    -1    -1    -1];

Fxyz = Fxyz.*sign_matrix; % convert to actuator local coordinate system.

== matlab function SixDsimulator_M1B/hp_chase ==
  data: Xm input; Xha output
function Xha = hp_chase(Xm)
% dm2dh is M1B to M1B
% convert to HP
Xha = -1e3*dm2dh(Xm);  % input to the mirror in mm
